simulink model "ESP_Model"  (R2021a)
settings: Solver=VariableStepAuto  StartTime=0.0  StopTime=4  MaxStep=.001  RelTol=1e-3
values from neighbouring files (symbols this model uses):
  A_brake_piston = 0.00369    [Vehicle_Dynamics.m]
  Af = 2    [Script.m]
  alpha = 0    [Script.m]    (also in Vehicle_Dynamics.m)
  Cd = 0.3    [Script.m]
  f = 0.01    [Script.m]    (also in Vehicle_Dynamics.m = 0.015)
  g = 9.81    [Script.m]    (also in Vehicle_Dynamics.m)
  h_g = 1.3    [Script.m]
  I = 1.2    [Script.m]
  iceDistance = 20    [Script.m]
  iceTime = 1.5    [Script.m]
  L = 5    [Script.m]
  l = 2.86258    [Vehicle_Dynamics.m]
  l_f = 1.226382    [Vehicle_Dynamics.m]
  l_r = l - l_f    (= 1.636198)    [Vehicle_Dynamics.m]
  Lr = 3    [Script.m]
  m = 1908    [Script.m]    (also in Vehicle_Dynamics.m = 1818)
  mu_brakepad = 0.5    [Vehicle_Dynamics.m]
  r = 0    [Vehicle_Dynamics.m]
  r_disc = 0.1405    [Vehicle_Dynamics.m]
  rho = 1.2    [Script.m]
  Rr = 0.767/2    (= 0.3835)    [Script.m]
  v0 = 90*1000/(60*60)    (= 25)    [Script.m]
  x0 = 0    [Script.m]
undefined symbols (not defined in the file or in its folder): brake, controller, h_s, sigbuilder_block, tire, wheel_diameter
libraries: pid_lib x6, simulink x5
(part 1 of 2)
settings Model: Creator=johnf  LastModifiedBy=johnf

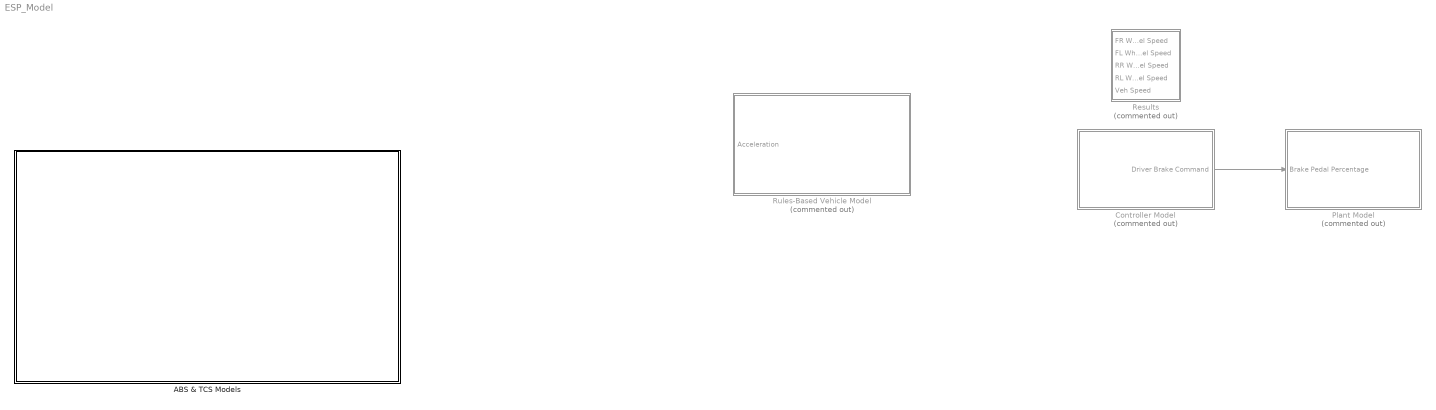
== system ESP_Model ==
  ABS & TCS Models : Subsystem
  Controller Model : Subsystem  Commented=on
  Plant Model : Subsystem  Commented=on
  Results : Subsystem  Commented=on
  Rules-Based Vehicle Model : Subsystem  Commented=on
  wires:
  Controller Model/1(Driver Brake Command) -> Plant Model/1(Brake Pedal Percentage)

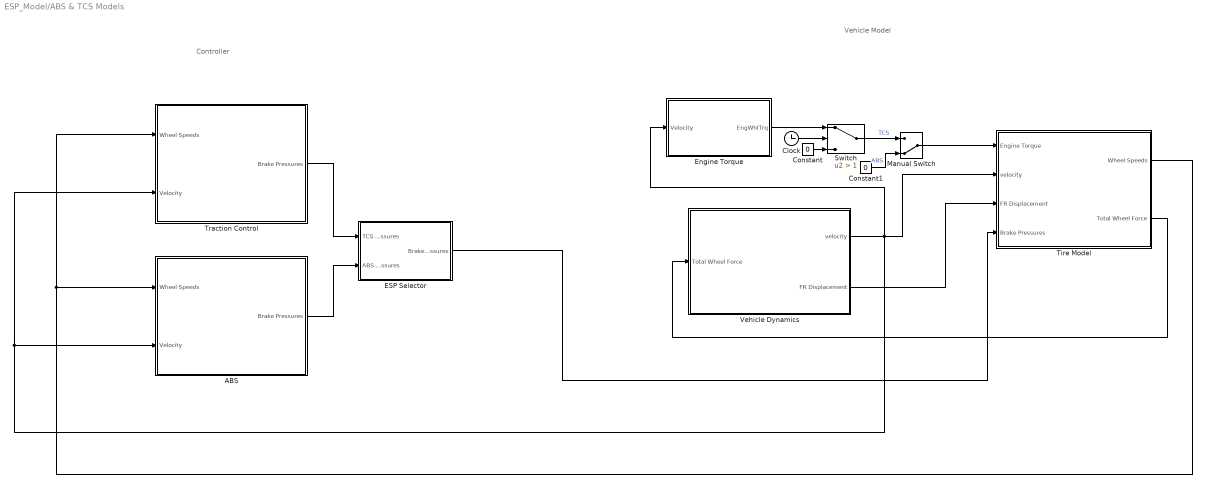
== system ESP_Model/ABS & TCS Models ==
  note: Vehicle Model
  note: Controller
  ABS : Subsystem
  Clock : Clock
  Constant : Constant  Value=0
  Constant1 : Constant  Value=0
  ESP Selector : Subsystem
  Engine Torque : Subsystem
  Manual Switch : ManualSwitch  CurrentSetting=0
  Switch : Switch  Criteria=u2 > Threshold  Threshold=1
  Tire Model : Subsystem
  Traction Control : Subsystem
  Vehicle Dynamics : Subsystem
  wires:
  Vehicle Dynamics/1(velocity) -> Engine Torque/1(Velocity), Traction Control/2(Velocity), ABS/2(Velocity), Tire Model/2(velocity)
  Constant1/1 -> Manual Switch/2  "ABS"
  Tire Model/1(Wheel Speeds) -> Traction Control/1(Wheel Speeds), ABS/1(Wheel Speeds)
  Manual Switch/1 -> Tire Model/1(Engine Torque)
  Tire Model/2(Total Wheel Force) -> Vehicle Dynamics/1(Total Wheel Force)
  Vehicle Dynamics/2(FR Displacement) -> Tire Model/3(FR Displacement)
  Traction Control/1(Brake Pressures) -> ESP Selector/1(TCS Pressures)
  ABS/1(Brake Pressures) -> ESP Selector/2(ABS Pressures)
  ESP Selector/1(Brake Pressures) -> Tire Model/4(Brake Pressures)
  Clock/1 -> Switch/2
  Constant/1 -> Switch/3
  Engine Torque/1(EngWhlTrq) -> Switch/1
  Switch/1 -> Manual Switch/1  "TCS"

== system ESP_Model/Controller Model ==
  Driver Commands : Subsystem
  Driver Brake Command : Outport
  wires:
  Driver Commands/1(Output) -> Driver Brake Command/1

== system ESP_Model/Plant Model ==
  Brake Pedal Percentage : Inport
  FR Brake : Subsystem
  Max Brake Pressure [PSI]1 : Gain  Gain=2000
  PSI to BAR1 : Gain  Gain=0.0689476
  wires:
  Max Brake Pressure [PSI]1/1 -> PSI to BAR1/1
  Brake Pedal Percentage/1 -> Max Brake Pressure [PSI]1/1
  PSI to BAR1/1 -> FR Brake/1(FR Brake Pressure from Driver)  "Master Cylinder Pressure"

== system ESP_Model/Results ==
  FR Wheel Speed : Inport
  FL Wheel Speed : Inport  Port=2
  RR Wheel Speed : Inport  Port=3
  RL Wheel Speed : Inport  Port=4
  Veh Speed : Inport  Port=5
  Vehicle Speed : Scope
  Wheel Speeds : Scope  NumInputPorts=4
  wires:
  FR Wheel Speed/1 -> Wheel Speeds/1
  FL Wheel Speed/1 -> Wheel Speeds/2
  RR Wheel Speed/1 -> Wheel Speeds/3
  RL Wheel Speed/1 -> Wheel Speeds/4
  Veh Speed/1 -> Vehicle Speed/1

== system ESP_Model/Rules-Based Vehicle Model ==
  Acceleration : Inport
  Braking Torque : Subsystem
  Dynamic Wheel Loads : Subsystem
  Integrator : Integrator  InitialCondition=90
  Slip Calculation : Subsystem
  Wheel Speeds : Subsystem
  wires:
  Acceleration/1 -> Integrator/1, Dynamic Wheel Loads/1(a_x)
  Integrator/1 -> Slip Calculation/2(Vehicle Speed), Wheel Speeds/1(Vehicle Speed)
  Wheel Speeds/1(Wheel Speed) -> Slip Calculation/1(Wheel Speed)

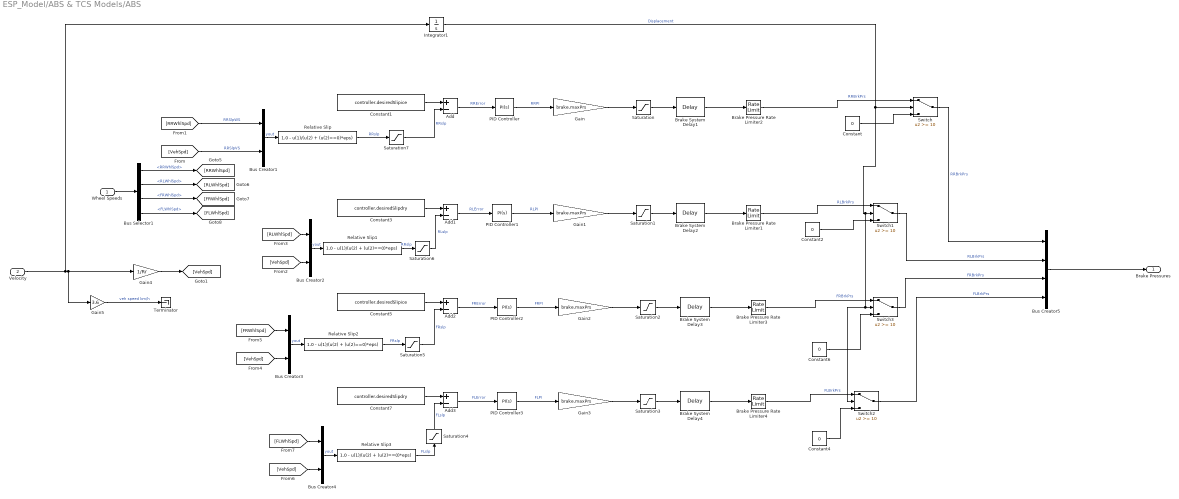
== system ESP_Model/ABS & TCS Models/ABS ==
  Wheel Speeds : Inport
  Velocity : Inport  Port=2
  Add{,1..3} (4 alike) : Sum  Inputs=+-
  Brake Pressure Rate Limiter{1..4} (4 alike) : RateLimiter  RisingSlewLimit=controller.slew  FallingSlewLimit=-controller.slew  SampleTimeMode=inherited
  Brake System Delay{1..4} (4 alike) : TransportDelay  DelayTime=controller.brkDelay
  Bus Creator5 : BusCreator  Inputs=4
  Bus Selector1 : BusSelector  OutputSignals=RRWhlSpd,RLWhlSpd,FRWhlSpd,FLWhlSpd
  Bus Creator{1..4} (4 alike) : BusCreator  Inputs=2
  Constant{,2,4,6} (4 alike) : Constant  Value=0
  Constant1 : Constant  Value=controller.desiredSlipice
  Constant3 : Constant  Value=controller.desiredSlipdry
  Constant5 : Constant  Value=controller.desiredSlipice
  Constant7 : Constant  Value=controller.desiredSlipdry
  Gain{,1..3} (4 alike) : Gain  Gain=brake.maxPrs
  Gain4 : Gain  Gain=1/Rr
  Gain5 : Gain  Gain=3.6
  Integrator1 : Integrator  InitialCondition=x0
  PID Controller : pid_lib/PID Controller  Controller=PI  Form=Parallel  TimeDomain=Continuous-time  UseExternalTs=off  SampleTime=-1  IntegratorMethod=Forward Euler  FilterMethod=Forward Euler  ControllerParametersSource=internal  P=0.5  I=1.4  D=0  UseFilter=on  N=100  TunerSelectOption=Transfer Function Based (PID Tuner App)  InitialConditionSource=internal  InitialConditionForIntegrator=1  InitialConditionForFilter=0  DifferentiatorICPrevScaledInput=0  ExternalReset=none  TrackingMode=off  Kt=1  LimitOutput=on  SatLimitsSource=internal  UpperSaturationLimit=1  LowerSaturationLimit=0  LinearizeAsGain=on  AntiWindupMode=none  Kb=1  POutMin=[]  POutMax=[]  IOutMin=[]  IOutMax=[]  DOutMin=[]  DOutMax=[]  NOutMin=[]  NOutMax=[]  SumOutMin=[]  SumOutMax=[]  SaturationOutMin=[]  SaturationOutMax=[]  PParamMin=[]  PParamMax=[]  IParamMin=[]  IParamMax=[]  DParamMin=[]  DParamMax=[]  NParamMin=[]  NParamMax=[]  KbParamMin=[]  KbParamMax=[]  KtParamMin=[]  KtParamMax=[]  KbOutMin=[]  KbOutMax=[]  KtOutMin=[]  KtOutMax=[]  IntegratorOutMin=[]  IntegratorOutMax=[]  FilterOutMin=[]  FilterOutMax=[]  SumI1OutMin=[]  SumI1OutMax=[]  SumI2OutMin=[]  SumI2OutMax=[]  SumI3OutMin=[]  SumI3OutMax=[]  SumI4OutMin=[]  SumI4OutMax=[]  SumDOutMin=[]  SumDOutMax=[]  DifferentiatorOutMin=[]  DifferentiatorOutMax=[]  FilterDiffOutCoefMin=[]  FilterDiffOutCoefMax=[]  ReciprocalOutMin=[]  ReciprocalOutMax=[]  SumDenOutMin=[]  SumDenOutMax=[]  SumNumOutMin=[]  SumNumOutMax=[]  DivideOutMin=[]  DivideOutMax=[]  UdiffTsProdOutMin=[]  UdiffTsProdOutMax=[]  NTsProdOutMin=[]  NTsProdOutMax=[]  UintegralTsProdOutMin=[]  UintegralTsProdOutMax=[]  UngainTsProdOutMin=[]  UngainTsProdOutMax=[]  IntegratorContinuousStateAttributes=''  IntegratorStateMustResolveToSignalObject=off  IntegratorRTWStateStorageClass=Auto  FilterContinuousStateAttributes=''  FilterStateMustResolveToSignalObject=off  FilterRTWStateStorageClass=Auto  ParallelPVariant=InternalParameters  IdealPVariant=Disabled  IVariant=InternalParameters  DVariant=Disabled  IntegratorVariant=Continuous  SatVariant=Enabled  AWVariant=Passthrough  PCopyVariant=Disabled  TRVariant=Disabled  FdbkBlocksVariant=Forward  IdealPFdbkVariant=Disabled  SatFdbkVariant=Disabled  DerivativeFilterVariant=Disabled  NVariant=Disabled  NCopyVariant=Disabled_SignalSpec  FilterICVariant=Disabled  IntegratorICVariant=InternalICs  ExternalResetVariant=Disabled  TRSumVariant=Passthrough  SumFdbkVariant=Disabled  SumVariant=Sum_PI  TsampFilterVariant=InternalTs  TsampNgainVariant=Passthrough  TsampIntegralVariant=Passthrough  ExternalSaturationOutDataTypeStr=Inherit: Same as second input
  PID Controller1 : pid_lib/PID Controller  Controller=PI  Form=Parallel  TimeDomain=Continuous-time  UseExternalTs=off  SampleTime=-1  IntegratorMethod=Forward Euler  FilterMethod=Forward Euler  ControllerParametersSource=internal  P=.5  I=1.4  D=0  UseFilter=on  N=100  TunerSelectOption=Transfer Function Based (PID Tuner App)  InitialConditionSource=internal  InitialConditionForIntegrator=1  InitialConditionForFilter=0  DifferentiatorICPrevScaledInput=0  ExternalReset=none  TrackingMode=off  Kt=1  LimitOutput=on  SatLimitsSource=internal  UpperSaturationLimit=1  LowerSaturationLimit=0  LinearizeAsGain=on  AntiWindupMode=none  Kb=1  POutMin=[]  POutMax=[]  IOutMin=[]  IOutMax=[]  DOutMin=[]  DOutMax=[]  NOutMin=[]  NOutMax=[]  SumOutMin=[]  SumOutMax=[]  SaturationOutMin=[]  SaturationOutMax=[]  PParamMin=[]  PParamMax=[]  IParamMin=[]  IParamMax=[]  DParamMin=[]  DParamMax=[]  NParamMin=[]  NParamMax=[]  KbParamMin=[]  KbParamMax=[]  KtParamMin=[]  KtParamMax=[]  KbOutMin=[]  KbOutMax=[]  KtOutMin=[]  KtOutMax=[]  IntegratorOutMin=[]  IntegratorOutMax=[]  FilterOutMin=[]  FilterOutMax=[]  SumI1OutMin=[]  SumI1OutMax=[]  SumI2OutMin=[]  SumI2OutMax=[]  SumI3OutMin=[]  SumI3OutMax=[]  SumI4OutMin=[]  SumI4OutMax=[]  SumDOutMin=[]  SumDOutMax=[]  DifferentiatorOutMin=[]  DifferentiatorOutMax=[]  FilterDiffOutCoefMin=[]  FilterDiffOutCoefMax=[]  ReciprocalOutMin=[]  ReciprocalOutMax=[]  SumDenOutMin=[]  SumDenOutMax=[]  SumNumOutMin=[]  SumNumOutMax=[]  DivideOutMin=[]  DivideOutMax=[]  UdiffTsProdOutMin=[]  UdiffTsProdOutMax=[]  NTsProdOutMin=[]  NTsProdOutMax=[]  UintegralTsProdOutMin=[]  UintegralTsProdOutMax=[]  UngainTsProdOutMin=[]  UngainTsProdOutMax=[]  IntegratorContinuousStateAttributes=''  IntegratorStateMustResolveToSignalObject=off  IntegratorRTWStateStorageClass=Auto  FilterContinuousStateAttributes=''  FilterStateMustResolveToSignalObject=off  FilterRTWStateStorageClass=Auto  ParallelPVariant=InternalParameters  IdealPVariant=Disabled  IVariant=InternalParameters  DVariant=Disabled  IntegratorVariant=Continuous  SatVariant=Enabled  AWVariant=Passthrough  PCopyVariant=Disabled  TRVariant=Disabled  FdbkBlocksVariant=Forward  IdealPFdbkVariant=Disabled  SatFdbkVariant=Disabled  DerivativeFilterVariant=Disabled  NVariant=Disabled  NCopyVariant=Disabled_SignalSpec  FilterICVariant=Disabled  IntegratorICVariant=InternalICs  ExternalResetVariant=Disabled  TRSumVariant=Passthrough  SumFdbkVariant=Disabled  SumVariant=Sum_PI  TsampFilterVariant=InternalTs  TsampNgainVariant=Passthrough  TsampIntegralVariant=Passthrough  ExternalSaturationOutDataTypeStr=Inherit: Same as second input
  PID Controller2 : pid_lib/PID Controller  Controller=PI  Form=Parallel  TimeDomain=Continuous-time  UseExternalTs=off  SampleTime=-1  IntegratorMethod=Forward Euler  FilterMethod=Forward Euler  ControllerParametersSource=internal  P=.5  I=1.4  D=0  UseFilter=on  N=100  TunerSelectOption=Transfer Function Based (PID Tuner App)  InitialConditionSource=internal  InitialConditionForIntegrator=1  InitialConditionForFilter=0  DifferentiatorICPrevScaledInput=0  ExternalReset=none  TrackingMode=off  Kt=1  LimitOutput=on  SatLimitsSource=internal  UpperSaturationLimit=1  LowerSaturationLimit=0  LinearizeAsGain=on  AntiWindupMode=none  Kb=1  POutMin=[]  POutMax=[]  IOutMin=[]  IOutMax=[]  DOutMin=[]  DOutMax=[]  NOutMin=[]  NOutMax=[]  SumOutMin=[]  SumOutMax=[]  SaturationOutMin=[]  SaturationOutMax=[]  PParamMin=[]  PParamMax=[]  IParamMin=[]  IParamMax=[]  DParamMin=[]  DParamMax=[]  NParamMin=[]  NParamMax=[]  KbParamMin=[]  KbParamMax=[]  KtParamMin=[]  KtParamMax=[]  KbOutMin=[]  KbOutMax=[]  KtOutMin=[]  KtOutMax=[]  IntegratorOutMin=[]  IntegratorOutMax=[]  FilterOutMin=[]  FilterOutMax=[]  SumI1OutMin=[]  SumI1OutMax=[]  SumI2OutMin=[]  SumI2OutMax=[]  SumI3OutMin=[]  SumI3OutMax=[]  SumI4OutMin=[]  SumI4OutMax=[]  SumDOutMin=[]  SumDOutMax=[]  DifferentiatorOutMin=[]  DifferentiatorOutMax=[]  FilterDiffOutCoefMin=[]  FilterDiffOutCoefMax=[]  ReciprocalOutMin=[]  ReciprocalOutMax=[]  SumDenOutMin=[]  SumDenOutMax=[]  SumNumOutMin=[]  SumNumOutMax=[]  DivideOutMin=[]  DivideOutMax=[]  UdiffTsProdOutMin=[]  UdiffTsProdOutMax=[]  NTsProdOutMin=[]  NTsProdOutMax=[]  UintegralTsProdOutMin=[]  UintegralTsProdOutMax=[]  UngainTsProdOutMin=[]  UngainTsProdOutMax=[]  IntegratorContinuousStateAttributes=''  IntegratorStateMustResolveToSignalObject=off  IntegratorRTWStateStorageClass=Auto  FilterContinuousStateAttributes=''  FilterStateMustResolveToSignalObject=off  FilterRTWStateStorageClass=Auto  ParallelPVariant=InternalParameters  IdealPVariant=Disabled  IVariant=InternalParameters  DVariant=Disabled  IntegratorVariant=Continuous  SatVariant=Enabled  AWVariant=Passthrough  PCopyVariant=Disabled  TRVariant=Disabled  FdbkBlocksVariant=Forward  IdealPFdbkVariant=Disabled  SatFdbkVariant=Disabled  DerivativeFilterVariant=Disabled  NVariant=Disabled  NCopyVariant=Disabled_SignalSpec  FilterICVariant=Disabled  IntegratorICVariant=InternalICs  ExternalResetVariant=Disabled  TRSumVariant=Passthrough  SumFdbkVariant=Disabled  SumVariant=Sum_PI  TsampFilterVariant=InternalTs  TsampNgainVariant=Passthrough  TsampIntegralVariant=Passthrough  ExternalSaturationOutDataTypeStr=Inherit: Same as second input
  PID Controller3 : pid_lib/PID Controller  Controller=PI  Form=Parallel  TimeDomain=Continuous-time  UseExternalTs=off  SampleTime=-1  IntegratorMethod=Forward Euler  FilterMethod=Forward Euler  ControllerParametersSource=internal  P=.5  I=1.4  D=0  UseFilter=on  N=100  TunerSelectOption=Transfer Function Based (PID Tuner App)  InitialConditionSource=internal  InitialConditionForIntegrator=1  InitialConditionForFilter=0  DifferentiatorICPrevScaledInput=0  ExternalReset=none  TrackingMode=off  Kt=1  LimitOutput=on  SatLimitsSource=internal  UpperSaturationLimit=1  LowerSaturationLimit=0  LinearizeAsGain=on  AntiWindupMode=none  Kb=1  POutMin=[]  POutMax=[]  IOutMin=[]  IOutMax=[]  DOutMin=[]  DOutMax=[]  NOutMin=[]  NOutMax=[]  SumOutMin=[]  SumOutMax=[]  SaturationOutMin=[]  SaturationOutMax=[]  PParamMin=[]  PParamMax=[]  IParamMin=[]  IParamMax=[]  DParamMin=[]  DParamMax=[]  NParamMin=[]  NParamMax=[]  KbParamMin=[]  KbParamMax=[]  KtParamMin=[]  KtParamMax=[]  KbOutMin=[]  KbOutMax=[]  KtOutMin=[]  KtOutMax=[]  IntegratorOutMin=[]  IntegratorOutMax=[]  FilterOutMin=[]  FilterOutMax=[]  SumI1OutMin=[]  SumI1OutMax=[]  SumI2OutMin=[]  SumI2OutMax=[]  SumI3OutMin=[]  SumI3OutMax=[]  SumI4OutMin=[]  SumI4OutMax=[]  SumDOutMin=[]  SumDOutMax=[]  DifferentiatorOutMin=[]  DifferentiatorOutMax=[]  FilterDiffOutCoefMin=[]  FilterDiffOutCoefMax=[]  ReciprocalOutMin=[]  ReciprocalOutMax=[]  SumDenOutMin=[]  SumDenOutMax=[]  SumNumOutMin=[]  SumNumOutMax=[]  DivideOutMin=[]  DivideOutMax=[]  UdiffTsProdOutMin=[]  UdiffTsProdOutMax=[]  NTsProdOutMin=[]  NTsProdOutMax=[]  UintegralTsProdOutMin=[]  UintegralTsProdOutMax=[]  UngainTsProdOutMin=[]  UngainTsProdOutMax=[]  IntegratorContinuousStateAttributes=''  IntegratorStateMustResolveToSignalObject=off  IntegratorRTWStateStorageClass=Auto  FilterContinuousStateAttributes=''  FilterStateMustResolveToSignalObject=off  FilterRTWStateStorageClass=Auto  ParallelPVariant=InternalParameters  IdealPVariant=Disabled  IVariant=InternalParameters  DVariant=Disabled  IntegratorVariant=Continuous  SatVariant=Enabled  AWVariant=Passthrough  PCopyVariant=Disabled  TRVariant=Disabled  FdbkBlocksVariant=Forward  IdealPFdbkVariant=Disabled  SatFdbkVariant=Disabled  DerivativeFilterVariant=Disabled  NVariant=Disabled  NCopyVariant=Disabled_SignalSpec  FilterICVariant=Disabled  IntegratorICVariant=InternalICs  ExternalResetVariant=Disabled  TRSumVariant=Passthrough  SumFdbkVariant=Disabled  SumVariant=Sum_PI  TsampFilterVariant=InternalTs  TsampNgainVariant=Passthrough  TsampIntegralVariant=Passthrough  ExternalSaturationOutDataTypeStr=Inherit: Same as second input
  Relative Slip{,1..3} (4 alike) : Fcn  Expr=1.0 - u(1)/(u(2) + (u(2)==0)*eps)
  Saturation{,1..3} (4 alike) : Saturate  UpperLimit=brake.maxPrs  LowerLimit=0
  Saturation{4..7} (4 alike) : Saturate  UpperLimit=1  LowerLimit=-1
  Switch{,1..3} (4 alike) : Switch  Threshold=10
  Terminator : Terminator
  Brake Pressures : Outport
  wires:
  Bus Creator1/1 -> Relative Slip/1  "yout"
  Relative Slip/1 -> Saturation7/1  "RRslp"
  Constant1/1 -> Add/1
  Add/1 -> PID Controller/1  "RRError"
  PID Controller/1 -> Gain/1  "RRPI"
  Gain/1 -> Saturation/1
  Saturation/1 -> Brake System Delay1/1
  Brake System Delay1/1 -> Brake Pressure Rate Limiter2/1
  Switch/1 -> Bus Creator5/1  "RRBrkPrs"
  [VehSpd] -> Bus Creator1/2  "RRSlpVS"
  [RRWhlSpd] -> Bus Creator1/1  "RRSlpWS"
  Constant3/1 -> Add1/1
  Bus Creator3/1 -> Relative Slip2/1  "yout"
  Relative Slip2/1 -> Saturation5/1  "FRslp"
  Constant5/1 -> Add2/1
  [VehSpd] -> Bus Creator3/2
  [FRWhlSpd] -> Bus Creator3/1
  [FLWhlSpd] -> Bus Creator4/1
  [VehSpd] -> Bus Creator4/2
  Constant7/1 -> Add3/1
  Saturation4/1 -> Add3/2  "FLslp"
  Bus Creator4/1 -> Relative Slip3/1  "yout"
  Relative Slip3/1 -> Saturation4/1  "FLslp"
  Saturation5/1 -> Add2/2  "FRslp"
  Saturation7/1 -> Add/2  "RRslp"
  Wheel Speeds/1 -> Bus Selector1/1
  Bus Selector1/4 -> [FLWhlSpd]  "<FLWhlSpd>"
  Bus Selector1/2 -> [RLWhlSpd]  "<RLWhlSpd>"
  Bus Selector1/1 -> [RRWhlSpd]  "<RRWhlSpd>"
  Bus Selector1/3 -> [FRWhlSpd]  "<FRWhlSpd>"
  PID Controller1/1 -> Gain1/1  "RLPI"
  Add1/1 -> PID Controller1/1  "RLError"
  Brake System Delay2/1 -> Brake Pressure Rate Limiter1/1
  Saturation1/1 -> Brake System Delay2/1
  Gain1/1 -> Saturation1/1
  Switch1/1 -> Bus Creator5/2  "RLBrkPrs"
  Switch3/1 -> Bus Creator5/3  "FRBrkPrs"
  Gain2/1 -> Saturation2/1
  Saturation2/1 -> Brake System Delay3/1
  Brake System Delay3/1 -> Brake Pressure Rate Limiter3/1
  Add2/1 -> PID Controller2/1  "FRError"
  PID Controller2/1 -> Gain2/1  "FRPI"
  Add3/1 -> PID Controller3/1  "FLError"
  PID Controller3/1 -> Gain3/1  "FLPI"
  Brake System Delay4/1 -> Brake Pressure Rate Limiter4/1
  Gain3/1 -> Saturation3/1
  Switch2/1 -> Bus Creator5/4  "FLBrkPrs"
  Saturation3/1 -> Brake System Delay4/1
  Saturation6/1 -> Add1/2  "RLslp"
  Relative Slip1/1 -> Saturation6/1  "RRslp"
  Bus Creator2/1 -> Relative Slip1/1  "yout"
  [RLWhlSpd] -> Bus Creator2/1
  [VehSpd] -> Bus Creator2/2
  Gain4/1 -> [VehSpd]
  Bus Creator5/1 -> Brake Pressures/1
  Velocity/1 -> Integrator1/1, Gain5/1, Gain4/1
  Gain5/1 -> Terminator/1  "veh speed km/h"
  Integrator1/1 -> Switch2/2, Switch3/2, Switch1/2, Switch/2  "Displacement"
  Brake Pressure Rate Limiter2/1 -> Switch/1  "RRBrkPrs"
  Constant/1 -> Switch/3
  Constant2/1 -> Switch1/3
  Constant4/1 -> Switch2/3
  Constant6/1 -> Switch3/3
  Brake Pressure Rate Limiter1/1 -> Switch1/1  "RLBrkPrs"
  Brake Pressure Rate Limiter3/1 -> Switch3/1  "FRBrkPrs"
  Brake Pressure Rate Limiter4/1 -> Switch2/1  "FLBrkPrs"

== system ESP_Model/ABS & TCS Models/ESP Selector ==
  TCS Pressures : Inport
  ABS Pressures : Inport  Port=2
  Bus Creator4 : BusCreator  Inputs=4
  Constant{11..14} (4 alike) : Constant  Value=brake.maxPrs
  Manual Switch1 : ManualSwitch  CurrentSetting=0
  Manual Switch2 : ManualSwitch
  Brake Pressures : Outport
  wires:
  ABS Pressures/1 -> Manual Switch1/2  "ABS"
  Manual Switch1/1 -> Manual Switch2/1
  TCS Pressures/1 -> Manual Switch1/1  "TCS"
  Constant11/1 -> Bus Creator4/4  "FLBrkPrs"
  Manual Switch2/1 -> Brake Pressures/1
  Constant12/1 -> Bus Creator4/3  "FRBrkPrs"
  Constant13/1 -> Bus Creator4/2  "RLBrkPrs"
  Constant14/1 -> Bus Creator4/1  "RRBrkPrs"
  Bus Creator4/1 -> Manual Switch2/2

== system ESP_Model/ABS & TCS Models/Engine Torque ==
  Velocity : Inport
  DiffGearRatio : Gain  Gain=2.77
  DiffSpdRatio : Gain  Gain=2.77
  Engine Torque vs Speed : Lookup_n-D  NumberOfTableDimensions=1  BreakpointsForDimension1=[500:500:5000]  Table=[200 250 350 350 340 325 275 250 225 200]  ExtrapMethod=Clip  UseLastTableValue=on  InternalRulePriority=Speed  RndMeth=Simplest  InputSameDT=on
  Gain1 : Gain  Gain=1/2
  TransGearRatio : Gain  Gain=3.1
  TransSpeedRatio : Gain  Gain=3.1
  m/s2rpm : Gain  Gain=60/(2*pi*Rr)
  EngWhlTrq : Outport  VectorParamsAs1DForOutWhenUnconnected=off
  wires:
  DiffGearRatio/1 -> Gain1/1  "EngWhlTrq"
  m/s2rpm/1 -> Engine Torque vs Speed/1  "EngRPM"
  DiffSpdRatio/1 -> TransSpeedRatio/1
  TransSpeedRatio/1 -> m/s2rpm/1
  Engine Torque vs Speed/1 -> TransGearRatio/1  "EngTorque"
  TransGearRatio/1 -> DiffGearRatio/1
  Velocity/1 -> DiffSpdRatio/1
  Gain1/1 -> EngWhlTrq/1

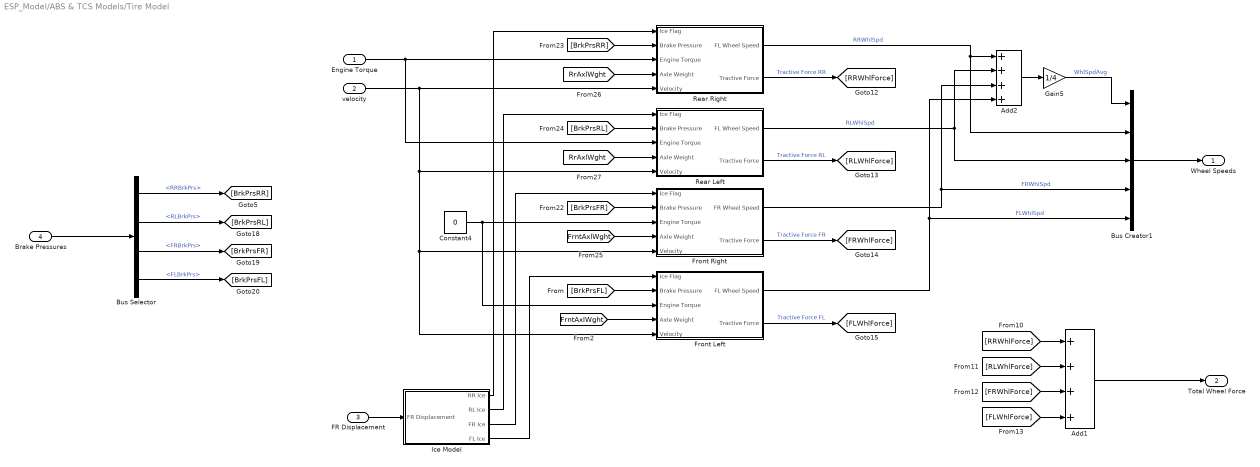
== system ESP_Model/ABS & TCS Models/Tire Model ==
  Engine Torque : Inport
  velocity : Inport  Port=2
  FR Displacement : Inport  Port=3
  Brake Pressures : Inport  Port=4
  Add1 : Sum  Inputs=++++
  Add2 : Sum  Inputs=4
  Bus Creator1 : BusCreator  Inputs=5
  Bus Selector : BusSelector  OutputSignals=RRBrkPrs,RLBrkPrs,FRBrkPrs,FLBrkPrs
  Constant4 : Constant  Value=0
  Front Left : Subsystem
  Front Right : Subsystem
  Gain5 : Gain  Gain=1/4
  Ice Model : Subsystem
  Rear Left : Subsystem
  Rear Right : Subsystem
  Wheel Speeds : Outport
  Total Wheel Force : Outport  Port=2
  wires:
  Front Right/2(Tractive Force) -> [FRWhlForce]  "Tractive Force FR"
  [FrntAxlWght] -> Front Left/4(Axle Weight)
  Ice Model/3(FR Ice) -> Front Right/1(Ice Flag)
  [BrkPrsFL] -> Front Left/2(Brake Pressure)
  [RrAxlWght] -> Rear Left/4(Axle Weight)
  Rear Right/2(Tractive Force) -> [RRWhlForce]  "Tractive Force RR"
  [BrkPrsFR] -> Front Right/2(Brake Pressure)
  velocity/1 -> Front Left/5(Velocity), Front Right/5(Velocity), Rear Left/5(Velocity), Rear Right/5(Velocity)
  Front Left/2(Tractive Force) -> [FLWhlForce]  "Tractive Force FL"
  Constant4/1 -> Front Left/3(Engine Torque), Front Right/3(Engine Torque)
  Ice Model/4(FL Ice) -> Front Left/1(Ice Flag)
  [BrkPrsRR] -> Rear Right/2(Brake Pressure)
  Ice Model/2(RL Ice) -> Rear Left/1(Ice Flag)
  [FrntAxlWght] -> Front Right/4(Axle Weight)
  [RrAxlWght] -> Rear Right/4(Axle Weight)
  [BrkPrsRL] -> Rear Left/2(Brake Pressure)
  Ice Model/1(RR Ice) -> Rear Right/1(Ice Flag)
  Rear Left/2(Tractive Force) -> [RLWhlForce]  "Tractive Force RL"
  Engine Torque/1 -> Rear Left/3(Engine Torque), Rear Right/3(Engine Torque)
  Gain5/1 -> Bus Creator1/1  "WhlSpdAvg"
  Bus Creator1/1 -> Wheel Speeds/1
  Add2/1 -> Gain5/1
  Front Right/1(FR Wheel Speed) -> Bus Creator1/4, Add2/3  "FRWhlSpd"
  Front Left/1(FL Wheel Speed) -> Bus Creator1/5, Add2/4  "FLWhlSpd"
  Rear Left/1(FL Wheel Speed) -> Bus Creator1/3, Add2/2  "RLWhlSpd"
  Rear Right/1(FL Wheel Speed) -> Add2/1, Bus Creator1/2  "RRWhlSpd"
  Add1/1 -> Total Wheel Force/1
  [FRWhlForce] -> Add1/3
  [RRWhlForce] -> Add1/1
  [FLWhlForce] -> Add1/4
  [RLWhlForce] -> Add1/2
  FR Displacement/1 -> Ice Model/1(FR Displacement)
  Bus Selector/1 -> [BrkPrsRR]  "<RRBrkPrs>"
  Bus Selector/2 -> [BrkPrsRL]  "<RLBrkPrs>"
  Bus Selector/3 -> [BrkPrsFR]  "<FRBrkPrs>"
  Bus Selector/4 -> [BrkPrsFL]  "<FLBrkPrs>"
  Brake Pressures/1 -> Bus Selector/1

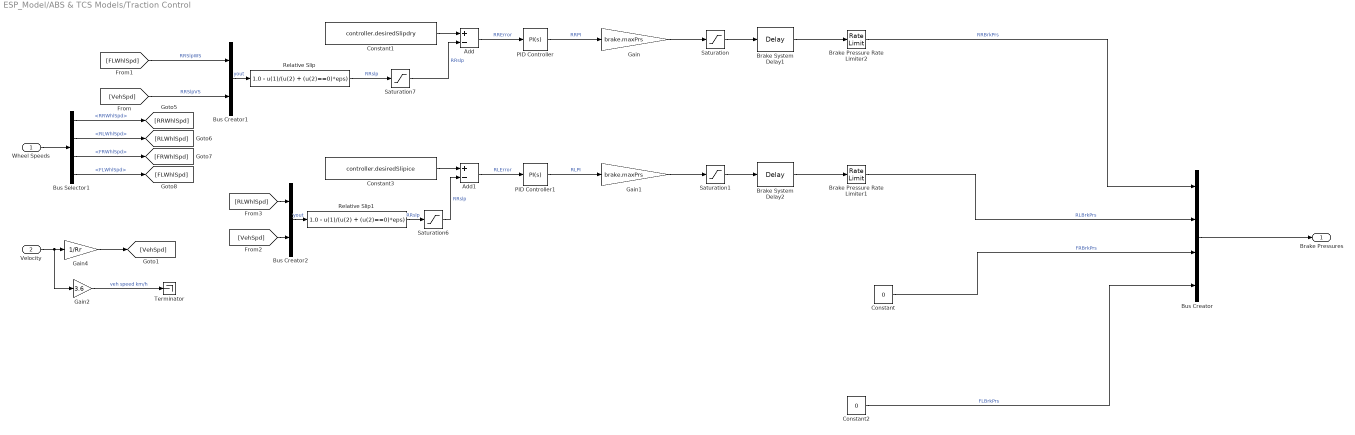
== system ESP_Model/ABS & TCS Models/Traction Control ==
  Wheel Speeds : Inport
  Velocity : Inport  Port=2
  Add : Sum  Inputs=+-
  Add1 : Sum  Inputs=+-
  Brake Pressure Rate Limiter1 : RateLimiter  RisingSlewLimit=controller.slew  FallingSlewLimit=-controller.slew  SampleTimeMode=inherited
  Brake Pressure Rate Limiter2 : RateLimiter  RisingSlewLimit=controller.slew  FallingSlewLimit=-controller.slew  SampleTimeMode=inherited
  Brake System Delay1 : TransportDelay  DelayTime=controller.brkDelay
  Brake System Delay2 : TransportDelay  DelayTime=controller.brkDelay
  Bus Creator : BusCreator  Inputs=4
  Bus Selector1 : BusSelector  OutputSignals=RRWhlSpd,RLWhlSpd,FRWhlSpd,FLWhlSpd
  Bus Creator1 : BusCreator  Inputs=2
  Bus Creator2 : BusCreator  Inputs=2
  Constant : Constant  Value=0
  Constant1 : Constant  Value=controller.desiredSlipdry
  Constant2 : Constant  Value=0
  Constant3 : Constant  Value=controller.desiredSlipice
  Gain : Gain  Gain=brake.maxPrs
  Gain1 : Gain  Gain=brake.maxPrs
  Gain2 : Gain  Gain=3.6
  Gain4 : Gain  Gain=1/Rr
  PID Controller : pid_lib/PID Controller  Controller=PI  Form=Parallel  TimeDomain=Continuous-time  UseExternalTs=off  SampleTime=-1  IntegratorMethod=Forward Euler  FilterMethod=Forward Euler  ControllerParametersSource=internal  P=0.2885  I=0.63  D=0  UseFilter=on  N=100  TunerSelectOption=Transfer Function Based (PID Tuner App)  InitialConditionSource=internal  InitialConditionForIntegrator=0  InitialConditionForFilter=0  DifferentiatorICPrevScaledInput=0  ExternalReset=none  TrackingMode=off  Kt=1  LimitOutput=on  SatLimitsSource=internal  UpperSaturationLimit=1  LowerSaturationLimit=0  LinearizeAsGain=on  AntiWindupMode=none  Kb=1  POutMin=[]  POutMax=[]  IOutMin=[]  IOutMax=[]  DOutMin=[]  DOutMax=[]  NOutMin=[]  NOutMax=[]  SumOutMin=[]  SumOutMax=[]  SaturationOutMin=[]  SaturationOutMax=[]  PParamMin=[]  PParamMax=[]  IParamMin=[]  IParamMax=[]  DParamMin=[]  DParamMax=[]  NParamMin=[]  NParamMax=[]  KbParamMin=[]  KbParamMax=[]  KtParamMin=[]  KtParamMax=[]  KbOutMin=[]  KbOutMax=[]  KtOutMin=[]  KtOutMax=[]  IntegratorOutMin=[]  IntegratorOutMax=[]  FilterOutMin=[]  FilterOutMax=[]  SumI1OutMin=[]  SumI1OutMax=[]  SumI2OutMin=[]  SumI2OutMax=[]  SumI3OutMin=[]  SumI3OutMax=[]  SumI4OutMin=[]  SumI4OutMax=[]  SumDOutMin=[]  SumDOutMax=[]  DifferentiatorOutMin=[]  DifferentiatorOutMax=[]  FilterDiffOutCoefMin=[]  FilterDiffOutCoefMax=[]  ReciprocalOutMin=[]  ReciprocalOutMax=[]  SumDenOutMin=[]  SumDenOutMax=[]  SumNumOutMin=[]  SumNumOutMax=[]  DivideOutMin=[]  DivideOutMax=[]  UdiffTsProdOutMin=[]  UdiffTsProdOutMax=[]  NTsProdOutMin=[]  NTsProdOutMax=[]  UintegralTsProdOutMin=[]  UintegralTsProdOutMax=[]  UngainTsProdOutMin=[]  UngainTsProdOutMax=[]  IntegratorContinuousStateAttributes=''  IntegratorStateMustResolveToSignalObject=off  IntegratorRTWStateStorageClass=Auto  FilterContinuousStateAttributes=''  FilterStateMustResolveToSignalObject=off  FilterRTWStateStorageClass=Auto  ParallelPVariant=InternalParameters  IdealPVariant=Disabled  IVariant=InternalParameters  DVariant=Disabled  IntegratorVariant=Continuous  SatVariant=Enabled  AWVariant=Passthrough  PCopyVariant=Disabled  TRVariant=Disabled  FdbkBlocksVariant=Forward  IdealPFdbkVariant=Disabled  SatFdbkVariant=Disabled  DerivativeFilterVariant=Disabled  NVariant=Disabled  NCopyVariant=Disabled_SignalSpec  FilterICVariant=Disabled  IntegratorICVariant=InternalICs  ExternalResetVariant=Disabled  TRSumVariant=Passthrough  SumFdbkVariant=Disabled  SumVariant=Sum_PI  TsampFilterVariant=InternalTs  TsampNgainVariant=Passthrough  TsampIntegralVariant=Passthrough  ExternalSaturationOutDataTypeStr=Inherit: Same as second input
  PID Controller1 : pid_lib/PID Controller  Controller=PI  Form=Parallel  TimeDomain=Continuous-time  UseExternalTs=off  SampleTime=-1  IntegratorMethod=Forward Euler  FilterMethod=Forward Euler  ControllerParametersSource=internal  P=0.2885  I=0.63  D=0  UseFilter=on  N=100  TunerSelectOption=Transfer Function Based (PID Tuner App)  InitialConditionSource=internal  InitialConditionForIntegrator=0  InitialConditionForFilter=0  DifferentiatorICPrevScaledInput=0  ExternalReset=none  TrackingMode=off  Kt=1  LimitOutput=on  SatLimitsSource=internal  UpperSaturationLimit=1  LowerSaturationLimit=0  LinearizeAsGain=on  AntiWindupMode=none  Kb=1  POutMin=[]  POutMax=[]  IOutMin=[]  IOutMax=[]  DOutMin=[]  DOutMax=[]  NOutMin=[]  NOutMax=[]  SumOutMin=[]  SumOutMax=[]  SaturationOutMin=[]  SaturationOutMax=[]  PParamMin=[]  PParamMax=[]  IParamMin=[]  IParamMax=[]  DParamMin=[]  DParamMax=[]  NParamMin=[]  NParamMax=[]  KbParamMin=[]  KbParamMax=[]  KtParamMin=[]  KtParamMax=[]  KbOutMin=[]  KbOutMax=[]  KtOutMin=[]  KtOutMax=[]  IntegratorOutMin=[]  IntegratorOutMax=[]  FilterOutMin=[]  FilterOutMax=[]  SumI1OutMin=[]  SumI1OutMax=[]  SumI2OutMin=[]  SumI2OutMax=[]  SumI3OutMin=[]  SumI3OutMax=[]  SumI4OutMin=[]  SumI4OutMax=[]  SumDOutMin=[]  SumDOutMax=[]  DifferentiatorOutMin=[]  DifferentiatorOutMax=[]  FilterDiffOutCoefMin=[]  FilterDiffOutCoefMax=[]  ReciprocalOutMin=[]  ReciprocalOutMax=[]  SumDenOutMin=[]  SumDenOutMax=[]  SumNumOutMin=[]  SumNumOutMax=[]  DivideOutMin=[]  DivideOutMax=[]  UdiffTsProdOutMin=[]  UdiffTsProdOutMax=[]  NTsProdOutMin=[]  NTsProdOutMax=[]  UintegralTsProdOutMin=[]  UintegralTsProdOutMax=[]  UngainTsProdOutMin=[]  UngainTsProdOutMax=[]  IntegratorContinuousStateAttributes=''  IntegratorStateMustResolveToSignalObject=off  IntegratorRTWStateStorageClass=Auto  FilterContinuousStateAttributes=''  FilterStateMustResolveToSignalObject=off  FilterRTWStateStorageClass=Auto  ParallelPVariant=InternalParameters  IdealPVariant=Disabled  IVariant=InternalParameters  DVariant=Disabled  IntegratorVariant=Continuous  SatVariant=Enabled  AWVariant=Passthrough  PCopyVariant=Disabled  TRVariant=Disabled  FdbkBlocksVariant=Forward  IdealPFdbkVariant=Disabled  SatFdbkVariant=Disabled  DerivativeFilterVariant=Disabled  NVariant=Disabled  NCopyVariant=Disabled_SignalSpec  FilterICVariant=Disabled  IntegratorICVariant=InternalICs  ExternalResetVariant=Disabled  TRSumVariant=Passthrough  SumFdbkVariant=Disabled  SumVariant=Sum_PI  TsampFilterVariant=InternalTs  TsampNgainVariant=Passthrough  TsampIntegralVariant=Passthrough  ExternalSaturationOutDataTypeStr=Inherit: Same as second input
  Relative Slip : Fcn  Expr=1.0 - u(1)/(u(2) + (u(2)==0)*eps)
  Relative Slip1 : Fcn  Expr=1.0 - u(1)/(u(2) + (u(2)==0)*eps)
  Saturation : Saturate  UpperLimit=brake.maxPrs  LowerLimit=0
  Saturation1 : Saturate  UpperLimit=brake.maxPrs  LowerLimit=0
  Saturation6 : Saturate  UpperLimit=1  LowerLimit=-1
  Saturation7 : Saturate  UpperLimit=1  LowerLimit=-1
  Terminator : Terminator
  Brake Pressures : Outport
  wires:
  Brake Pressure Rate Limiter2/1 -> Bus Creator/1  "RRBrkPrs"
  Constant3/1 -> Add1/1
  Wheel Speeds/1 -> Bus Selector1/1
  Bus Selector1/4 -> [FLWhlSpd]  "<FLWhlSpd>"
  Bus Selector1/2 -> [RLWhlSpd]  "<RLWhlSpd>"
  Bus Selector1/1 -> [RRWhlSpd]  "<RRWhlSpd>"
  Bus Selector1/3 -> [FRWhlSpd]  "<FRWhlSpd>"
  PID Controller1/1 -> Gain1/1  "RLPI"
  Add1/1 -> PID Controller1/1  "RLError"
  Brake System Delay2/1 -> Brake Pressure Rate Limiter1/1
  Saturation1/1 -> Brake System Delay2/1
  Gain1/1 -> Saturation1/1
  Brake Pressure Rate Limiter1/1 -> Bus Creator/2  "RLBrkPrs"
  Saturation6/1 -> Add1/2  "RRslp"
  Relative Slip1/1 -> Saturation6/1  "RRslp"
  Bus Creator2/1 -> Relative Slip1/1  "yout"
  [RLWhlSpd] -> Bus Creator2/1
  [VehSpd] -> Bus Creator2/2
  Velocity/1 -> Gain2/1, Gain4/1
  Gain4/1 -> [VehSpd]
  Constant/1 -> Bus Creator/3  "FRBrkPrs"
  Constant2/1 -> Bus Creator/4  "FLBrkPrs"
  Bus Creator/1 -> Brake Pressures/1
  Bus Creator1/1 -> Relative Slip/1  "yout"
  Add/1 -> PID Controller/1  "RRError"
  [VehSpd] -> Bus Creator1/2  "RRSlpVS"
  Gain/1 -> Saturation/1
  Brake System Delay1/1 -> Brake Pressure Rate Limiter2/1
  Constant1/1 -> Add/1
  Saturation7/1 -> Add/2  "RRslp"
  [FLWhlSpd] -> Bus Creator1/1  "RRSlpWS"
  Saturation/1 -> Brake System Delay1/1
  Relative Slip/1 -> Saturation7/1  "RRslp"
  PID Controller/1 -> Gain/1  "RRPI"
  Gain2/1 -> Terminator/1  "veh speed km/h"

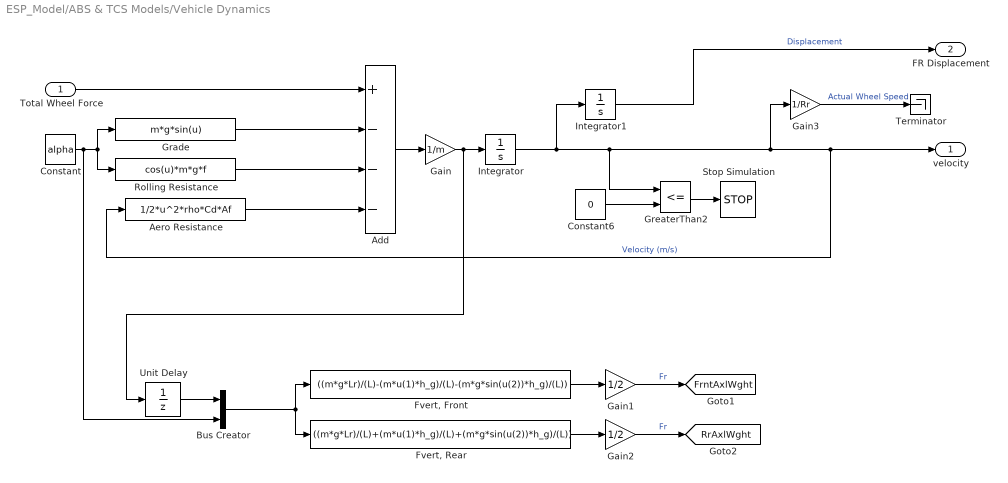
== system ESP_Model/ABS & TCS Models/Vehicle Dynamics ==
  Total Wheel Force : Inport
  Add : Sum  Inputs=+---
  Aero Resistance : Fcn  Expr=1/2*u^2*rho*Cd*Af
  Bus Creator : BusCreator  Inputs=2
  Constant : Constant  Value=alpha
  Constant6 : Constant  Value=0
  "Fvert, Front" : Fcn  Expr=((m*g*Lr)/(L)-(m*u(1)*h_g)/(L)-(m*g*sin(u(2))*h_g)/(L))
  "Fvert, Rear" : Fcn  Expr=((m*g*Lr)/(L)+(m*u(1)*h_g)/(L)+(m*g*sin(u(2))*h_g)/(L))
  Gain : Gain  Gain=1/m
  Gain1 : Gain  Gain=1/2
  Gain2 : Gain  Gain=1/2
  Gain3 : Gain  Gain=1/Rr
  Grade : Fcn  Expr=m*g*sin(u)
  GreaterThan2 : RelationalOperator  Operator=<=  OutDataTypeStr=boolean  RndMeth=Simplest
  Integrator : Integrator  InitialCondition=v0
  Integrator1 : Integrator  InitialCondition=x0
  Rolling Resistance : Fcn  Expr=cos(u)*m*g*f
  Stop Simulation : Stop
  Terminator : Terminator
  Unit Delay : UnitDelay  SampleTime=-1  HasFrameUpgradeWarning=on
  velocity : Outport
  FR Displacement : Outport  Port=2
  tag scope: FrntAxlWght=global, RrAxlWght=global
  wires:
  Grade/1 -> Add/2
  Rolling Resistance/1 -> Add/3
  GreaterThan2/1 -> Stop Simulation/1
  Add/1 -> Gain/1
  "Fvert, Front"/1 -> Gain1/1
  Integrator/1 -> Integrator1/1, GreaterThan2/1, Gain3/1, Aero Resistance/1, velocity/1  "Velocity (m/s)"
  Constant/1 -> Bus Creator/2, Rolling Resistance/1, Grade/1
  Constant6/1 -> GreaterThan2/2
  Integrator1/1 -> FR Displacement/1  "Displacement"
  Gain1/1 -> [FrntAxlWght]  "Fr"
  Bus Creator/1 -> "Fvert, Rear"/1, "Fvert, Front"/1
  Gain3/1 -> Terminator/1  "Actual Wheel Speed"
  Gain2/1 -> [RrAxlWght]  "Fr"
  Total Wheel Force/1 -> Add/1
  Unit Delay/1 -> Bus Creator/1
  Aero Resistance/1 -> Add/4
  "Fvert, Rear"/1 -> Gain2/1
  Gain/1 -> Unit Delay/1, Integrator/1

== system ESP_Model/Controller Model/Driver Commands ==
  Driver-Applied Brake Pedal Percentage : Subsystem  Tag=STV Subsys  LoadFcn=sigbuilder_block('load');  StartFcn=sigbuilder_block('start');  StopFcn=sigbuilder_block('stop');  ClipboardFcn=sigbuilder_block('clipboard');  mask(Sigbuilder block){tuvar=[0:10]}
      mask help: Simulink:masks:SigbuilderBlock_MD
      mask init:
      | if ~strcmp(get_param(bdroot(gcbh),'SimulationStatus'),'stopped') tuvar = sigbuilder_block('maskInit'); end
      settings: CopyFcn=sigbuilder_block('copy');  DeleteFcn=sigbuilder_block('delete');  ModelCloseFcn=sigbuilder_block('modelClose');  PreSaveFcn=sigbuilder_block('preSave');  PauseFcn=sigbuilder_block('pause');  ContinueFcn=sigbuilder_block('continue');  NameChangeFcn=sigbuilder_block('namechange');  OpenFcn=sigbuilder_block('open',[437.6 199.2 550.4 400 ]);  CloseFcn=sigbuilder_block('close');
      mask Display: plot(0, 0, 100, 100,[2, 2, 32, 32, 2], [68, 8, 8, 68, 68],[32, 2], [38, 38], [32, 19, 2],[53, 60, 44], [32, 17, 17, 2],[16, 16, 31, 31]);txt = getActiveGroup(gcbh);text(2, 100, txt,'verticalAlignment', 'top');
  Output : Outport
  wires:
  Driver-Applied Brake Pedal Percentage/1(Signal 1) -> Output/1

== system ESP_Model/Plant Model/FR Brake ==
  note: Integrates Brake Pressure Dynamic value [bar/s]
      | from assignment to get pressure [bar]
  note: Stops reducing brake pressure
      | once output brake pressure is zero
  note: Only reduces brake pressure
      | if driver applies brake
  FR Brake Pressure from Driver : Inport
  Add : Sum  Inputs=++-
  Constant : Constant  Value=100
  Constant1 : Constant  Value=0
  Constant2 : Constant  Value=0
  Integrator : Integrator
  Saturation Dynamic : simulink/Discontinuities/Saturation Dynamic  OutMin=[]  OutMax=[]  OutDataTypeStr=Inherit: Same as second input  OutDataType=fixdt(1, 16)  OutScaling=2^-10  DoSatur=off
  Scope : Scope
  Switch : Switch  Criteria=u2 > Threshold
  Switch1 : Switch
  wires:
  Constant1/1 -> Switch/3
  Constant2/1 -> Switch1/3
  Switch/1 -> Switch1/1
  Switch1/1 -> Integrator/1
  Add/1 -> Switch1/2, Add/1, Scope/1  "Ouput"
  FR Brake Pressure from Driver/1 -> Add/2, Switch/2  "Master Cylinder Pressure"
  Integrator/1 -> Add/3  "Accumulator Pressure"
  Constant/1 -> Switch/1

== system ESP_Model/Rules-Based Vehicle Model/Braking Torque ==
  note: Pressure in Bar
  Brake On/Off : Inport
  Constant : Constant  Value=96
  Constant1 : Constant  Value=A_brake_piston
  Constant2 : Constant  Value=mu_brakepad
  Constant3 : Constant  Value=r_disc
  Product : Product  Inputs=4
  Product1 : Product
  Rate Limiter : RateLimiter  RisingSlewLimit=100  FallingSlewLimit=-100  SampleTimeMode=inherited
  Braking Torque : Outport
  wires:
  Constant1/1 -> Product/2
  Constant2/1 -> Product/3
  Constant3/1 -> Product/4
  Product/1 -> Braking Torque/1
  Rate Limiter/1 -> Product/1
  Product1/1 -> Rate Limiter/1
  Constant/1 -> Product1/1
  Brake On/Off/1 -> Product1/2

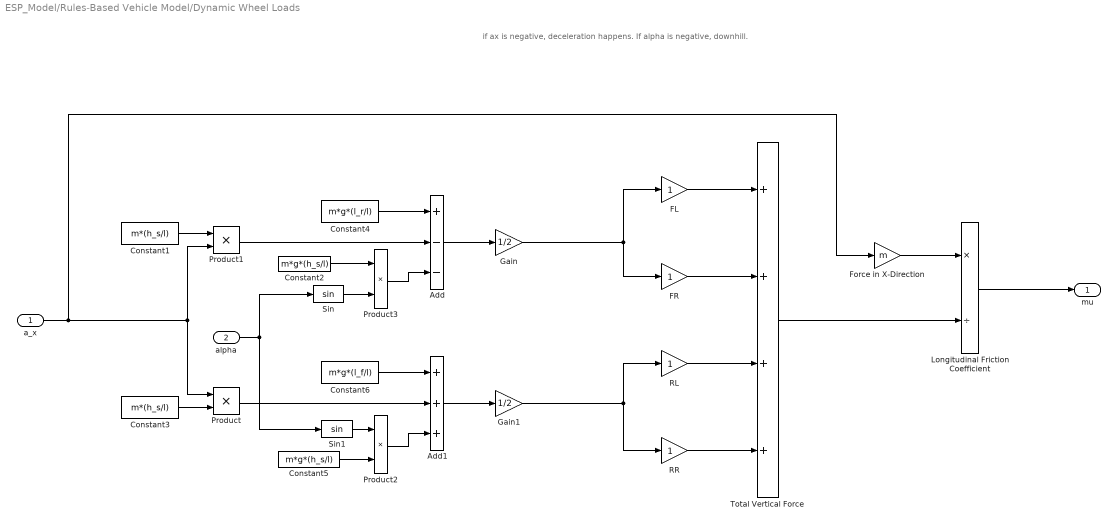
== system ESP_Model/Rules-Based Vehicle Model/Dynamic Wheel Loads ==
  note: if ax is negative, deceleration happens. If alpha is negative, downhill.
  a_x : Inport
  alpha : Inport  Port=2
  Add : Sum  Inputs=+--
  Add1 : Sum  Inputs=+++
  Constant1 : Constant  Value=m*(h_s/l)
  Constant2 : Constant  Value=m*g*(h_s/l)
  Constant3 : Constant  Value=m*(h_s/l)
  Constant4 : Constant  Value=m*g*(l_r/l)
  Constant5 : Constant  Value=m*g*(h_s/l)
  Constant6 : Constant  Value=m*g*(l_f/l)
  FL : Gain
  FR : Gain
  Force in X-Direction : Gain  Gain=m
  Gain : Gain  Gain=1/2
  Gain1 : Gain  Gain=1/2
  Longitudinal Friction Coefficient : Product  Inputs=*/
  Product{,1..3} (4 alike) : Product
  RL : Gain
  RR : Gain
  Sin : Trigonometry
  Sin1 : Trigonometry
  Total Vertical Force : Sum  Inputs=++++
  mu : Outport
  wires:
  Constant6/1 -> Add1/1
  Add1/1 -> Gain1/1
  Gain1/1 -> RR/1, RL/1
  Gain/1 -> FL/1, FR/1
  Add/1 -> Gain/1
  Constant4/1 -> Add/1
  FL/1 -> Total Vertical Force/1
  FR/1 -> Total Vertical Force/2
  RL/1 -> Total Vertical Force/3
  RR/1 -> Total Vertical Force/4
  Total Vertical Force/1 -> Longitudinal Friction Coefficient/2
  Force in X-Direction/1 -> Longitudinal Friction Coefficient/1
  Product/1 -> Add1/2
  Constant3/1 -> Product/2
  a_x/1 -> Force in X-Direction/1, Product1/2, Product/1
  Constant1/1 -> Product1/1
  Product1/1 -> Add/2
  alpha/1 -> Sin1/1, Sin/1
  Sin/1 -> Product3/2
  Sin1/1 -> Product2/1
  Product3/1 -> Add/3
  Constant2/1 -> Product3/1
  Product2/1 -> Add1/3
  Constant5/1 -> Product2/2
  Longitudinal Friction Coefficient/1 -> mu/1

== system ESP_Model/Rules-Based Vehicle Model/Slip Calculation ==
  Wheel Speed : Inport
  Vehicle Speed : Inport  Port=2
  Add : Sum  Inputs=+-
  Divide : Product  Inputs=*/
  Gain : Gain  Gain=r
  Slip : Outport
  wires:
  Wheel Speed/1 -> Gain/1
  Gain/1 -> Add/2
  Vehicle Speed/1 -> Add/1, Divide/2
  Add/1 -> Divide/1
  Divide/1 -> Slip/1

== system ESP_Model/Rules-Based Vehicle Model/Wheel Speeds ==
  Vehicle Speed : Inport
  m/s to RPM : Gain  Gain=60/(wheel_diameter*pi)
  Wheel Speed : Outport
  wires:
  m/s to RPM/1 -> Wheel Speed/1
  Vehicle Speed/1 -> m/s to RPM/1

== system ESP_Model/ABS & TCS Models/Tire Model/Front Left ==
  Ice Flag : Inport
  Brake Pressure : Inport  Port=2
  Engine Torque : Inport  Port=3
  Axle Weight : Inport  Port=4
  Velocity : Inport  Port=5
  FL : Subsystem
  Slip Model Dry : Subsystem
  Slip Model Ice : Subsystem
  Switch1 : Switch  Threshold=1
  FL Wheel Speed : Outport  VectorParamsAs1DForOutWhenUnconnected=off
  Tractive Force : Outport  Port=2  VectorParamsAs1DForOutWhenUnconnected=off
  wires:
  Ice Flag/1 -> Switch1/2
  FL/1(WheelSpeed) -> Slip Model Dry/2(WheelSpeed (rad/s)), Slip Model Ice/2(WheelSpeed (rad/s)), FL Wheel Speed/1
  Slip Model Dry/1(mu) -> Switch1/3
  Brake Pressure/1 -> FL/2(Brake Pressure)
  Slip Model Ice/1(mu) -> Switch1/1
  Engine Torque/1 -> FL/3(Engine Torque)
  Axle Weight/1 -> FL/4(weight)
  FL/2(AxleF) -> Tractive Force/1
  Velocity/1 -> Slip Model Dry/1(VehVel (m/s)), Slip Model Ice/1(VehVel (m/s))
  Switch1/1 -> FL/1(frictionCoefficient)

== system ESP_Model/ABS & TCS Models/Tire Model/Front Right ==
  Ice Flag : Inport
  Brake Pressure : Inport  Port=2
  Engine Torque : Inport  Port=3
  Axle Weight : Inport  Port=4
  Velocity : Inport  Port=5
  Fr : Subsystem
  Slip Model Dry : Subsystem
  Slip Model Ice : Subsystem
  Switch1 : Switch  Threshold=1
  FR Wheel Speed : Outport  VectorParamsAs1DForOutWhenUnconnected=off
  Tractive Force : Outport  Port=2  VectorParamsAs1DForOutWhenUnconnected=off
  wires:
  Switch1/1 -> Fr/1(frictionCoefficient)
  Velocity/1 -> Slip Model Dry/1(VehVel (m/s)), Slip Model Ice/1(VehVel (m/s))
  Fr/2(AxleF) -> Tractive Force/1
  Axle Weight/1 -> Fr/4(weight)
  Engine Torque/1 -> Fr/3(Engine Torque)
  Slip Model Ice/1(mu) -> Switch1/1
  Brake Pressure/1 -> Fr/2(Brake Pressure)
  Slip Model Dry/1(mu) -> Switch1/3
  Fr/1(WheelSpeed) -> Slip Model Dry/2(WheelSpeed (rad/s)), Slip Model Ice/2(WheelSpeed (rad/s)), FR Wheel Speed/1
  Ice Flag/1 -> Switch1/2

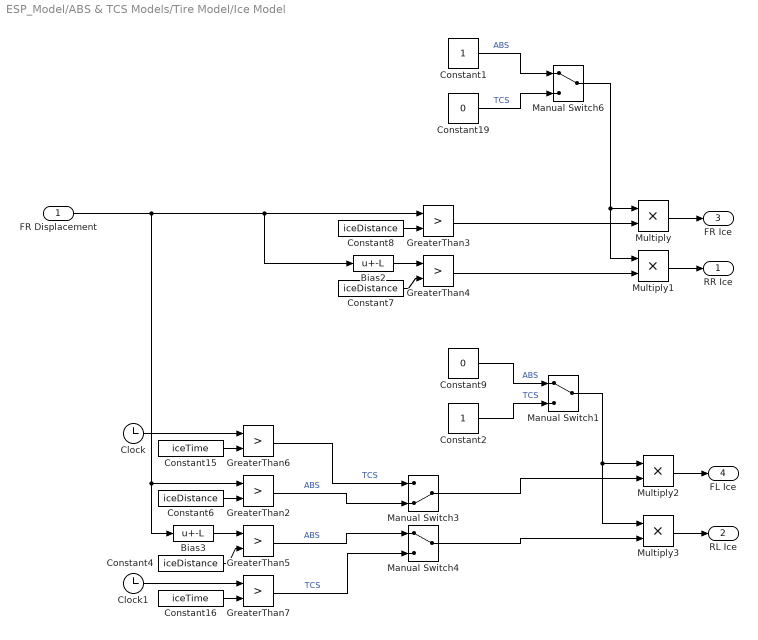
== system ESP_Model/ABS & TCS Models/Tire Model/Ice Model ==
  FR Displacement : Inport
  Bias2 : Bias  Bias=-L
  Bias3 : Bias  Bias=-L
  Clock : Clock
  Clock1 : Clock
  Constant1 : Constant
  Constant15 : Constant  Value=iceTime
  Constant16 : Constant  Value=iceTime
  Constant19 : Constant  Value=0
  Constant2 : Constant
  Constant{4,6..8} (4 alike) : Constant  Value=iceDistance
  Constant9 : Constant  Value=0
  GreaterThan{2..7} (6 alike) : RelationalOperator  Operator=>  OutDataTypeStr=boolean  RndMeth=Simplest
  Manual Switch1 : ManualSwitch
  Manual Switch3 : ManualSwitch  CurrentSetting=0
  Manual Switch4 : ManualSwitch
  Manual Switch6 : ManualSwitch
  Multiply{,1..3} (4 alike) : Product
  RR Ice : Outport
  RL Ice : Outport  Port=2
  FR Ice : Outport  Port=3
  FL Ice : Outport  Port=4
  wires:
  Constant7/1 -> GreaterThan4/2
  Bias2/1 -> GreaterThan4/1
  Manual Switch6/1 -> Multiply1/1, Multiply/1
  Multiply/1 -> FR Ice/1
  Multiply1/1 -> RR Ice/1
  GreaterThan4/1 -> Multiply1/2
  Manual Switch1/1 -> Multiply2/1, Multiply3/1
  Multiply3/1 -> RL Ice/1
  GreaterThan3/1 -> Multiply/2
  Constant8/1 -> GreaterThan3/2
  Multiply2/1 -> FL Ice/1
  Constant19/1 -> Manual Switch6/2  "TCS"
  Constant1/1 -> Manual Switch6/1  "ABS"
  Constant2/1 -> Manual Switch1/2  "TCS"
  Constant9/1 -> Manual Switch1/1  "ABS"
  Constant16/1 -> GreaterThan7/2
  Clock1/1 -> GreaterThan7/1
  GreaterThan6/1 -> Manual Switch3/1  "TCS"
  Clock/1 -> GreaterThan6/1
  GreaterThan7/1 -> Manual Switch4/2  "TCS"
  FR Displacement/1 -> Bias2/1, GreaterThan3/1, GreaterThan2/1, Bias3/1
  GreaterThan2/1 -> Manual Switch3/2  "ABS"
  Constant4/1 -> GreaterThan5/2
  GreaterThan5/1 -> Manual Switch4/1  "ABS"
  Constant6/1 -> GreaterThan2/2
  Constant15/1 -> GreaterThan6/2
  Bias3/1 -> GreaterThan5/1
  Manual Switch3/1 -> Multiply2/2
  Manual Switch4/1 -> Multiply3/2

== system ESP_Model/ABS & TCS Models/Tire Model/Rear Left ==
  Ice Flag : Inport
  Brake Pressure : Inport  Port=2
  Engine Torque : Inport  Port=3
  Axle Weight : Inport  Port=4
  Velocity : Inport  Port=5
  Fr : Subsystem
  Slip Model Dry : Subsystem
  Slip Model Ice : Subsystem
  Switch1 : Switch  Threshold=1
  FL Wheel Speed : Outport  VectorParamsAs1DForOutWhenUnconnected=off
  Tractive Force : Outport  Port=2  VectorParamsAs1DForOutWhenUnconnected=off
  wires:
  Ice Flag/1 -> Switch1/2
  Fr/1(WheelSpeed) -> Slip Model Dry/2(WheelSpeed (rad/s)), Slip Model Ice/2(WheelSpeed (rad/s)), FL Wheel Speed/1  "FL Wheel Speed"
  Slip Model Dry/1(mu) -> Switch1/3
  Brake Pressure/1 -> Fr/2(Brake Pressure)
  Slip Model Ice/1(mu) -> Switch1/1
  Engine Torque/1 -> Fr/3(Engine Torque)
  Axle Weight/1 -> Fr/4(weight)
  Fr/2(AxleF) -> Tractive Force/1
  Velocity/1 -> Slip Model Ice/1(VehVel (m/s)), Slip Model Dry/1(VehVel (m/s))
  Switch1/1 -> Fr/1(frictionCoefficient)

== system ESP_Model/ABS & TCS Models/Tire Model/Rear Right ==
  Ice Flag : Inport
  Brake Pressure : Inport  Port=2
  Engine Torque : Inport  Port=3
  Axle Weight : Inport  Port=4
  Velocity : Inport  Port=5
  Fr1 : Subsystem
  Slip Model Dry : Subsystem
  Slip Model Ice : Subsystem
  Switch1 : Switch  Threshold=1
  FL Wheel Speed : Outport  VectorParamsAs1DForOutWhenUnconnected=off
  Tractive Force : Outport  Port=2  VectorParamsAs1DForOutWhenUnconnected=off
  wires:
  Switch1/1 -> Fr1/1(frictionCoefficient)
  Velocity/1 -> Slip Model Ice/1(VehVel (m/s)), Slip Model Dry/1(VehVel (m/s))
  Fr1/2(AxleF) -> Tractive Force/1
  Axle Weight/1 -> Fr1/4(weight)
  Engine Torque/1 -> Fr1/3(Engine Torque)
  Slip Model Ice/1(mu) -> Switch1/1
  Brake Pressure/1 -> Fr1/2(Brake Pressure)
  Slip Model Dry/1(mu) -> Switch1/3
  Fr1/1(WheelSpeed) -> Slip Model Dry/2(WheelSpeed (rad/s)), Slip Model Ice/2(WheelSpeed (rad/s)), FL Wheel Speed/1
  Ice Flag/1 -> Switch1/2

== system ESP_Model/Controller Model/Driver Commands/Driver-Applied Brake Pedal Percentage ==
  Demux : Demux  Tag=STV Demux  Outputs=1
      settings: DisplayOption=none
  FromWs : FromWorkspace  Tag=STV FromWs  VariableName=tuvar
      SigBuilderData=|
      | common.afterFinalStr = 'Extrapolate'
      | common.sampleTime = 0
      | dataSet.timeRange = [0 10]
      | dataSet.name = 'Group 1'
      | sbobj.Groups.Name = 'Group 1'
      | sbobj.Groups.Signals.Name = 'Signal 1'
      | sbobj.Groups.Signals.XData = [0 4 4 10]
      | sbobj.Groups.Signals.YData = [0 0 1.01 1.01]
  Signal 1 : Outport  Tag=STV Outport
  wires:
  Demux/1 -> Signal 1/1
  FromWs/1 -> Demux/1

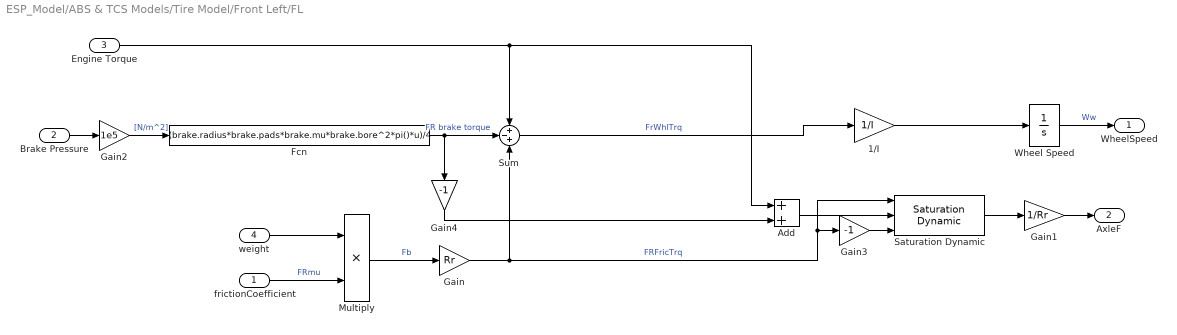
== system ESP_Model/ABS & TCS Models/Tire Model/Front Left/FL ==
  frictionCoefficient : Inport
  Brake Pressure : Inport  Port=2
  Engine Torque : Inport  Port=3
  weight : Inport  Port=4
  1/I : Gain  Gain=1/I  SaturateOnIntegerOverflow=on  OutDataTypeStr=Inherit: Same as input  ParamDataTypeStr=Inherit: Same as input
  Add : Sum
  Fcn : Fcn  Expr=(brake.radius*brake.pads*brake.mu*brake.bore^2*pi()*u)/4
  Gain : Gain  Gain=Rr
  Gain1 : Gain  Gain=1/Rr
  Gain2 : Gain  Gain=1e5
  Gain3 : Gain  Gain=-1
  Gain4 : Gain  Gain=-1
  Multiply : Product
  Saturation Dynamic : simulink/Discontinuities/Saturation Dynamic  OutMin=[]  OutMax=[]  OutDataTypeStr=Inherit: Same as second input  OutDataType=fixdt(1, 16)  OutScaling=2^-10  DoSatur=off
  Sum : Sum  Inputs=+-+  InputSameDT=on  SaturateOnIntegerOverflow=on  OutDataTypeStr=Inherit: Same as first input
  Wheel Speed : Integrator  InitialCondition=v0/Rr  LimitOutput=on  UpperSaturationLimit=1000  LowerSaturationLimit=0
  WheelSpeed : Outport  VectorParamsAs1DForOutWhenUnconnected=off
  AxleF : Outport  Port=2  VectorParamsAs1DForOutWhenUnconnected=off
  wires:
  Engine Torque/1 -> Sum/1, Add/1
  1/I/1 -> Wheel Speed/1
  Brake Pressure/1 -> Gain2/1
  Fcn/1 -> Gain4/1, Sum/2  "FR brake torque"
  Wheel Speed/1 -> WheelSpeed/1  "Ww"
  weight/1 -> Multiply/1
  frictionCoefficient/1 -> Multiply/2  "FRmu"
  Multiply/1 -> Gain/1  "Fb"
  Gain/1 -> Sum/3, Saturation Dynamic/1, Gain3/1  "FRFricTrq"
  Gain1/1 -> AxleF/1
  Gain2/1 -> Fcn/1  "[N/m^2]"
  Saturation Dynamic/1 -> Gain1/1
  Gain3/1 -> Saturation Dynamic/3
  Gain4/1 -> Add/2
  Add/1 -> Saturation Dynamic/2
  Sum/1 -> 1/I/1  "FrWhlTrq"

== system ESP_Model/ABS & TCS Models/Tire Model/Front Left/Slip Model Dry ==
  VehVel (m/s) : Inport
  WheelSpeed (rad/s) : Inport  Port=2
  Bus Creator : BusCreator  Inputs=2
  Gain : Gain  Gain=1/Rr
  Relative Slip : Fcn  Expr=1.0 - u(1)/(u(2) + (u(2)==0)*eps)
  dry : Fcn  Expr=tire.dry(3)*sin(tire.dry(2)*atan((tire.dry(1)*u(1))-(tire.dry(4)*((tire.dry(1)*u(1))-atan(tire.dry(1)*u(1))))))
  mu : Outport  VectorParamsAs1DForOutWhenUnconnected=off
  wires:
  Relative Slip/1 -> dry/1  "slp"
  Bus Creator/1 -> Relative Slip/1  "yout"
  dry/1 -> mu/1
  WheelSpeed (rad/s)/1 -> Bus Creator/1
  VehVel (m/s)/1 -> Gain/1
  Gain/1 -> Bus Creator/2

== system ESP_Model/ABS & TCS Models/Tire Model/Front Left/Slip Model Ice ==
  VehVel (m/s) : Inport
  WheelSpeed (rad/s) : Inport  Port=2
  Bus Creator : BusCreator  Inputs=2
  Gain : Gain  Gain=1/Rr
  Relative Slip : Fcn  Expr=1.0 - u(1)/(u(2) + (u(2)==0)*eps)
  ice : Fcn  Expr=tire.ice(3)*sin(tire.ice(2)*atan((tire.ice(1)*u(1))-(tire.ice(4)*((tire.ice(1)*u(1))-atan(tire.ice(1)*u(1))))))
  mu : Outport  VectorParamsAs1DForOutWhenUnconnected=off
  wires:
  WheelSpeed (rad/s)/1 -> Bus Creator/1
  ice/1 -> mu/1
  Bus Creator/1 -> Relative Slip/1  "yout"
  Relative Slip/1 -> ice/1  "slp"
  VehVel (m/s)/1 -> Gain/1
  Gain/1 -> Bus Creator/2

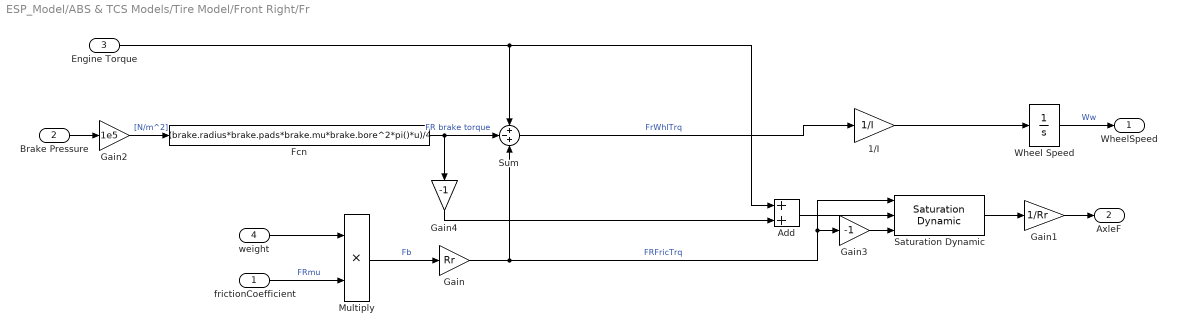
== system ESP_Model/ABS & TCS Models/Tire Model/Front Right/Fr ==
  frictionCoefficient : Inport
  Brake Pressure : Inport  Port=2
  Engine Torque : Inport  Port=3
  weight : Inport  Port=4
  1/I : Gain  Gain=1/I  SaturateOnIntegerOverflow=on  OutDataTypeStr=Inherit: Same as input  ParamDataTypeStr=Inherit: Same as input
  Add : Sum
  Fcn : Fcn  Expr=(brake.radius*brake.pads*brake.mu*brake.bore^2*pi()*u)/4
  Gain : Gain  Gain=Rr
  Gain1 : Gain  Gain=1/Rr
  Gain2 : Gain  Gain=1e5
  Gain3 : Gain  Gain=-1
  Gain4 : Gain  Gain=-1
  Multiply : Product
  Saturation Dynamic : simulink/Discontinuities/Saturation Dynamic  OutMin=[]  OutMax=[]  OutDataTypeStr=Inherit: Same as second input  OutDataType=fixdt(1, 16)  OutScaling=2^-10  DoSatur=off
  Sum : Sum  Inputs=+-+  InputSameDT=on  SaturateOnIntegerOverflow=on  OutDataTypeStr=Inherit: Same as first input
  Wheel Speed : Integrator  InitialCondition=v0/Rr  LimitOutput=on  UpperSaturationLimit=1000  LowerSaturationLimit=0
  WheelSpeed : Outport  VectorParamsAs1DForOutWhenUnconnected=off
  AxleF : Outport  Port=2  VectorParamsAs1DForOutWhenUnconnected=off
  wires:
  Engine Torque/1 -> Sum/1, Add/1
  1/I/1 -> Wheel Speed/1
  Brake Pressure/1 -> Gain2/1
  Fcn/1 -> Gain4/1, Sum/2  "FR brake torque"
  Wheel Speed/1 -> WheelSpeed/1  "Ww"
  weight/1 -> Multiply/1
  frictionCoefficient/1 -> Multiply/2  "FRmu"
  Multiply/1 -> Gain/1  "Fb"
  Gain/1 -> Sum/3, Saturation Dynamic/1, Gain3/1  "FRFricTrq"
  Gain1/1 -> AxleF/1
  Gain2/1 -> Fcn/1  "[N/m^2]"
  Saturation Dynamic/1 -> Gain1/1
  Gain3/1 -> Saturation Dynamic/3
  Gain4/1 -> Add/2
  Add/1 -> Saturation Dynamic/2
  Sum/1 -> 1/I/1  "FrWhlTrq"

== system ESP_Model/ABS & TCS Models/Tire Model/Front Right/Slip Model Dry ==
  VehVel (m/s) : Inport
  WheelSpeed (rad/s) : Inport  Port=2
  Bus Creator : BusCreator  Inputs=2
  Gain : Gain  Gain=1/Rr
  Relative Slip : Fcn  Expr=1.0 - u(1)/(u(2) + (u(2)==0)*eps)
  dry : Fcn  Expr=tire.dry(3)*sin(tire.dry(2)*atan((tire.dry(1)*u(1))-(tire.dry(4)*((tire.dry(1)*u(1))-atan(tire.dry(1)*u(1))))))
  mu : Outport  VectorParamsAs1DForOutWhenUnconnected=off
  wires:
  Relative Slip/1 -> dry/1  "slp"
  Bus Creator/1 -> Relative Slip/1  "yout"
  dry/1 -> mu/1
  WheelSpeed (rad/s)/1 -> Bus Creator/1
  VehVel (m/s)/1 -> Gain/1
  Gain/1 -> Bus Creator/2

== system ESP_Model/ABS & TCS Models/Tire Model/Front Right/Slip Model Ice ==
  VehVel (m/s) : Inport
  WheelSpeed (rad/s) : Inport  Port=2
  Bus Creator : BusCreator  Inputs=2
  Gain : Gain  Gain=1/Rr
  Relative Slip : Fcn  Expr=1.0 - u(1)/(u(2) + (u(2)==0)*eps)
  ice : Fcn  Expr=tire.ice(3)*sin(tire.ice(2)*atan((tire.ice(1)*u(1))-(tire.ice(4)*((tire.ice(1)*u(1))-atan(tire.ice(1)*u(1))))))
  mu : Outport  VectorParamsAs1DForOutWhenUnconnected=off
  wires:
  WheelSpeed (rad/s)/1 -> Bus Creator/1
  ice/1 -> mu/1
  Bus Creator/1 -> Relative Slip/1  "yout"
  Relative Slip/1 -> ice/1  "slp"
  Gain/1 -> Bus Creator/2
  VehVel (m/s)/1 -> Gain/1
